simulink model "cl"  (R2017a)
settings: Solver=VariableStepAuto  StartTime=0.0  StopTime=40  RelTol=1e-3
settings Model: Creator=Mr.li  LastModifiedBy=Mr.li

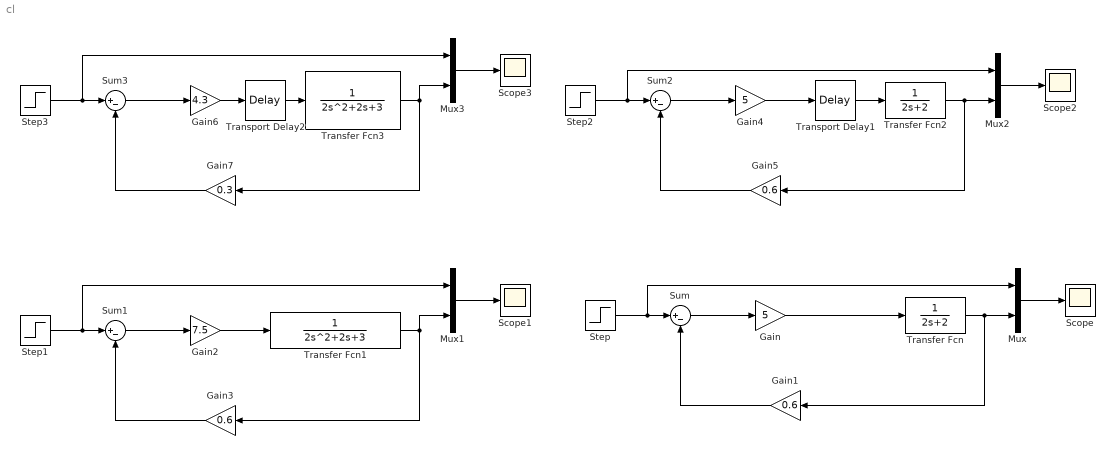
== system cl ==
  Gain : Gain  Gain=5
  Gain1 : Gain  Gain=0.6
  Gain2 : Gain  Gain=7.5
  Gain3 : Gain  Gain=0.6
  Gain4 : Gain  Gain=5
  Gain5 : Gain  Gain=0.6
  Gain6 : Gain  Gain=4.3
  Gain7 : Gain  Gain=0.3
  Mux{,1..3} (4 alike) : Mux  Inputs=2
  Scope{,1..3} (4 alike) : Scope
  Step{,1..3} (4 alike) : Step  SampleTime=0
  Sum{,1..3} (4 alike) : Sum  Inputs=|+-
  Transfer Fcn : TransferFcn  Denominator=[2 2]
  Transfer Fcn1 : TransferFcn  Denominator=[2 2 3]
  Transfer Fcn2 : TransferFcn  Denominator=[2 2]
  Transfer Fcn3 : TransferFcn  Denominator=[2 2 3]
  Transport Delay1 : TransportDelay
  Transport Delay2 : TransportDelay
  wires:
  Step/1 -> Mux/1, Sum/1
  Sum/1 -> Gain/1
  Mux/1 -> Scope/1
  Gain1/1 -> Sum/2
  Transfer Fcn/1 -> Gain1/1, Mux/2
  Mux1/1 -> Scope1/1
  Gain3/1 -> Sum1/2
  Sum1/1 -> Gain2/1
  Step1/1 -> Mux1/1, Sum1/1
  Transfer Fcn1/1 -> Gain3/1, Mux1/2
  Gain2/1 -> Transfer Fcn1/1
  Transport Delay1/1 -> Transfer Fcn2/1
  Mux2/1 -> Scope2/1
  Gain5/1 -> Sum2/2
  Gain4/1 -> Transport Delay1/1
  Sum2/1 -> Gain4/1
  Step2/1 -> Mux2/1, Sum2/1
  Transfer Fcn2/1 -> Gain5/1, Mux2/2
  Transport Delay2/1 -> Transfer Fcn3/1
  Mux3/1 -> Scope3/1
  Gain7/1 -> Sum3/2
  Gain6/1 -> Transport Delay2/1
  Sum3/1 -> Gain6/1
  Step3/1 -> Mux3/1, Sum3/1
  Transfer Fcn3/1 -> Gain7/1, Mux3/2
  Gain/1 -> Transfer Fcn/1
